simulink model "BasicTransferFunction"  (R2013a)
settings: Solver=ode45  StartTime=0.0  StopTime=10.0  RelTol=1e-3
settings Model: Creator=stuart  LastModifiedBy=stuart

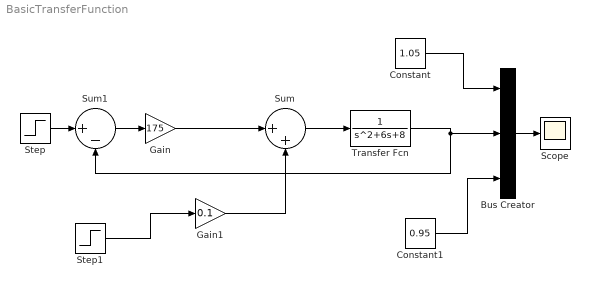
== system BasicTransferFunction ==
  Bus Creator : BusCreator  Inputs=3
  Constant : Constant  Value=1.05
  Constant1 : Constant  Value=0.95
  Gain : Gain  Gain=175
  Gain1 : Gain  Gain=0.1
  Scope : Scope
  Step : Step  Time=0  SampleTime=0
  Step1 : Step  Time=0  SampleTime=0
  Sum : Sum  Inputs=|++
  Sum1 : Sum  Inputs=|+-
  Transfer Fcn : TransferFcn  Denominator=[1 6 8]
  wires:
  Step/1 -> Sum1/1
  Gain/1 -> Sum/1
  Sum/1 -> Transfer Fcn/1
  Step1/1 -> Gain1/1
  Gain1/1 -> Sum/2
  Sum1/1 -> Gain/1
  Transfer Fcn/1 -> Sum1/2, Bus Creator/2
  Bus Creator/1 -> Scope/1
  Constant1/1 -> Bus Creator/3
  Constant/1 -> Bus Creator/1
